simulink model "predictive_continuous_simulation_20241118_2015b"  (R2015b)
settings: Solver=ode4  SolverMode=SingleTasking  StartTime=0.0  StopTime=Tend  FixedStep=Ts  MaxStep=Ts  MinStep=Ts  RelTol=1e-3
values from neighbouring files (symbols this model uses):
  gamma = 2    [code_simu.m]    (also in code_simu_continuous_simplified.m = 100000; matlab.mat = 1000)
  sigma = 10    [code_simu.m]    (also in code_simu_continuous_simplified.m = 0.01; matlab.mat = 100)
undefined symbols (not defined in the file or in its folder): ae, Afp, As, bap_bar, bap_v, be, beta0, beta1, beta2, bfp, cap_bar, den_filter, dena0, denf, denp, exp_cap2, fn, M1, M3, M3_v_2, M4_v_2, M_bar, num_filter, numa0, numf, nump, Pf, r, setpoint, setpoint_time, sin_f, T, T_gairan, Tf, Tf_n, Tf_n_vec, Tref, Ts, tstf_vec, v_max, YM
(part 2 of 2)

== matlab function predictive_continuous_simulation_20241118_2015b/Predictive_controller1/Subsystem3/MATLAB Function1 ==
  data: ym input; ep input; z2_hat input; v output; cap_bar input; beta0 input; Tf_n input; Ts input; Tf input; tstf_vec input; lamuda_0 input; x_ap input; M3_v_2 parameter; M4_v_2 parameter; As parameter; bap_v parameter; T parameter; exp_cap2 parameter
function v = fcn(ym,ep,z2_hat,cap_bar,beta0,Tf_n,Ts,Tf,tstf_vec,lamuda_0,x_ap,M3_v_2, M4_v_2,As,bap_v,T,exp_cap2)
%#codegen
% aa,ba,Afp,bfp,r,Pf,T
%     Aap_bar = [aa zeros(1,length(Afp)); zeros(length(Afp),1) Afp];
%     bap_bar = [ba;bfp];
%     As = [Aap_bar -bap_bar*bap_bar.'/r; -cap_bar*cap_bar.' -Aap_bar.'];
% 
% M3_v = zeros(length(As)/2,length(As)/2,length(tstf_vec));
% M4_v = zeros(length(As)/2,length(As)/2,length(tstf_vec));
%   for j = 0:Ts:Tf 
%     M = expm(As*(j));                    
% %     M1 = M(1:length(M)/2 , 1:length(M)/2);
% %     M2 = M(1:length(M)/2 , length(M)/2+1:length(M));
%     M3 = M(length(M)/2+1:length(M) , 1:length(M)/2);
%     M4 = M(length(M)/2+1:length(M) , length(M)/2+1:length(M));
%     
%     M3_v(:,:,round(1+j/Ts)) = M3;
%     M4_v(:,:,round(1+j/Ts)) = M4;
%     
%     % M_bar = inv([M4-Pf*M2 -cap_bar; cap_bar.'*M2 0]);  
%     
%         
%   end
%   bap_v = -bap_bar.'/r; 
 %%%--------------------------------------------------------------------%%
 %%%--------------------------------------------------------------------%%
 
a_vec = zeros(length(cap_bar)*2,length(tstf_vec));
a_vec_int = zeros(length(cap_bar)*2,1);

%%%  tf-t0
%%% ∫     exp(As*tau)*tr([0 ca_bar])*ym(tf-tau)*dtau
%%%  0
%%% 台形積分を使用
%%% サンプリング時間ごとの，0からt-t0までの被積分関数値を計算 
a2_vec = zeros(length(cap_bar),length(tstf_vec));
    ii=1;
    for i = 0:Ts:Tf
%         a_vec(:,round(1+i/Ts)) = exp_cap2(:,:,ii)*[z2_hat;ym(round(Tf_n+1-i/Ts))]; 
        a_vec(:,round(1+i/Ts)) = exp_cap2(:,:,ii)*[z2_hat-beta0*ep;ym(round(Tf_n+1-i/Ts))];
        ii=ii+1;
    end
%%% 台形積分
    for i = 1:length(As)
        a_vec_int(i,1) = trapz(tstf_vec,a_vec(i,:));
    end
   for j = 0:Ts:Tf           % j が時刻 t 
%     for i = 0:Ts:j
%         a_vec(:,round(1+i/Ts)) = expm(As*i)*[[1;zeros(length(cap_bar)-1,1)] zeros(length(cap_bar),1); zeros(length(cap_bar),1) cap_bar]*[z2_hat-beta0*ep;ym(round(Tf_n+1-i/Ts))]; 
%     end
% %%% 台形積分
%     for i = 1:length(As)
%         a_vec_int(i,1) = trapz(tstf_vec,a_vec(i,:));
%     end
   
        % a1_vec = a_vec_int(1:length(cap_bar));
        a2_vec(:,round(1+j/Ts)) = a_vec_int(length(cap_bar)+1:length(cap_bar)*2);
   end
 %%%--------------------------------------------------------------------%%
 %%%--------------------------------------------------------------------%%

   v_bar = zeros(1,Tf/Ts+1); % 1+Tf/Ts
    for j = 0:Ts:Tf
     lamuda = M3_v_2(:,:,round(1+j/Ts))*x_ap + M4_v_2(:,:,round(1+j/Ts))*lamuda_0 + a2_vec(:,round(1+j/Ts));
     v_bar(1,round(1+j/Ts)) = bap_v*lamuda;
    end
    
%      v = v_bar(1:round(1+T/Ts));  %%%
   
     v = v_bar(1+T/Ts);  % T/Ts
%      v = v_bar(1);  % T/Ts

== matlab function predictive_continuous_simulation_20241118_2015b/Subsystem2/in_out4 ==
  data: setpoint output; t input; setpoint_vec input; t_num output; setpoint_time input; count input
function [setpoint,t_num]  = fcn(t,setpoint_vec,setpoint_time,count)
%#codegen
%%% 目標値の生成

count_n = count;

if(count_n<=length(setpoint_time) && t>=setpoint_time(int8(count_n)) && t~=0)
    count_n = count_n+1;
end

setpoint = setpoint_vec(int8(count_n));

t_num = count_n;

== matlab function predictive_continuous_simulation_20241118_2015b/Subsystem2/in_out5 ==
  data: setpoint input; Tref input; Tf_n_vec input; Ts input; ym_out output; ym1 input; ym_in output
function [ym_out,ym_in]   = fcn(setpoint,Tref,Tf_n_vec,Ts,ym1)
%#codegen
%%% 規範信号の生成
%%% 現時刻:ym(t) から 現時刻＋予測時間:ym(t+Tf) まで

nym = length(Tf_n_vec)+1;

ym = zeros(1,nym);
ym(1) = ym1;
    for k = 2:nym
        ym(1,k) = setpoint - exp(-Ts/Tref)*(setpoint-ym(1,k-1));
    end
ym_out = ym;
ym_in = ym(2);

== matlab function predictive_continuous_simulation_20241118_2015b/Subsystem3/in_out4 ==
  data: setpoint output; t input; setpoint_vec input; t_num output; setpoint_time input; count input
function [setpoint,t_num]  = fcn(t,setpoint_vec,setpoint_time,count)
%#codegen
%%% 目標値の生成

count_n = count;

if(count_n<=length(setpoint_time) && t>=setpoint_time(int8(count_n)) && t~=0)
    count_n = count_n+1;
end

setpoint = setpoint_vec(int8(count_n));

t_num = count_n;

== matlab function predictive_continuous_simulation_20241118_2015b/Subsystem3/in_out5 ==
  data: setpoint input; Tref input; Tf_n_vec input; Ts input; ym_out output; ym1 input; ym_in output
function [ym_out,ym_in]   = fcn(setpoint,Tref,Tf_n_vec,Ts,ym1)
%#codegen
%%% 規範信号の生成
%%% 現時刻:ym(t) から 現時刻＋予測時間:ym(t+Tf) まで

nym = length(Tf_n_vec)+1;

ym = zeros(1,nym);
ym(1) = ym1;
    for k = 2:nym
        ym(1,k) = setpoint - exp(-Ts/Tref)*(setpoint-ym(1,k-1));
    end
ym_out = ym;
ym_in = ym(2);

== matlab function predictive_continuous_simulation_20241118_2015b/future signal1/MATLAB Function ==
  data: u input; Tf_n_vec input; ym output; u_in input
function ym = fcn(u,Tf_n_vec,u_in)


a = length(Tf_n_vec);
ym = zeros(1,a + 1);
ym(1,1:a) = u_in(1,2:a+1);
ym(1,a+1) = u;

== matlab function predictive_continuous_simulation_20241118_2015b/in_out2 ==
  data: in input; out output
function out = fcn(in)
%#codegen
out = in(1,1);

== matlab function predictive_continuous_simulation_20241118_2015b/ym_sin1/MATLAB Function ==
  data: Tf_n_vec input; ym output; t input; Ts input; omega_sin input
function ym = fcn(Tf_n_vec,t,Ts,omega_sin)
a = length(Tf_n_vec)+1

ym = zeros(1,a)
for i = 1:a
    ym(i) = sin(2*pi*omega_sin*(t+(i-1)*Ts))+0.5;
end
